simulink model "STM32"  (R2019b)
settings: Solver=FixedStepAuto  StartTime=0.0  StopTime=5  RelTol=1e-3  EnableMultiTasking=on
undefined symbols (not defined in the file): DiscIntNeverNeededParam
libraries: simulink x2, eePwmGenerator x1, pspsim x1
settings Model: SILPILModeSetting=veronly  ExtModeTrigDuration=10  Creator=ahmet  LastModifiedBy=ahmet
settings SolverCC: AlgebraicLoopSolver=LineSearch  PositivePriorityOrder=on  AutoInsertRateTranBlk=on
settings OptimizationCC: EnhancedBackFolding=on  PassReuseOutputArgsAs=Individual arguments  ZeroExternalMemoryAtStartup=off  ZeroInternalMemoryAtStartup=off  MaxStackSize=64  OptimizeBlockOrder=speed  DifferentSizesBufferReuse=on  OptimizationCustomize=off  EfficientTunableParamExpr=on
settings DebuggingCC: AlgebraicLoopMsg=none  ParameterTunabilityLossMsg=error
settings HardwareCC: ProdBitPerPointer=32  ProdBitPerSizeT=32  ProdBitPerPtrDiffT=32  ProdLargestAtomicInteger=Long  ProdLargestAtomicFloat=Double  ProdWordSize=32  ProdHWDeviceType=ARM Compatible->ARM Cortex
settings ModelReferenceCC: ModelReferenceNumInstancesAllowed=Single
settings SFSimCC: MATLABDynamicMemAlloc=off
settings RTWCC: SystemTargetFile=ert.tlc  HardwareBoard=STM32F4-Discovery  TLCOptions="-aInlineSetEventsForThisBaseRateFcn=TLC_FALSE -aSuppressMultiTaskScheduler=TLC_FALSE   -aRateBasedStepFcn=1"  TemplateMakefile=ert_default_tmf  GenerateReport=on  Toolchain=GNU Tools for ARM Embedded Processors  IncludeHyperlinkInReport=on  LaunchReport=on  GenerateTraceInfo=on  GenerateTraceReport=on  GenerateTraceReportSl=on  GenerateTraceReportSf=on  GenerateTraceReportEml=on
settings CodeAppCC: ForceParamTrailComments=on  IgnoreCustomStorageClasses=off  OperatorAnnotations=on  SimulinkDataObjDesc=on  SFDataObjDesc=on  InsertBlockDesc=on
settings ERTTargetCC: CodeReplacementLibrary=ARM Cortex-M (Optimized)  ExtModeStaticAllocSize=2000

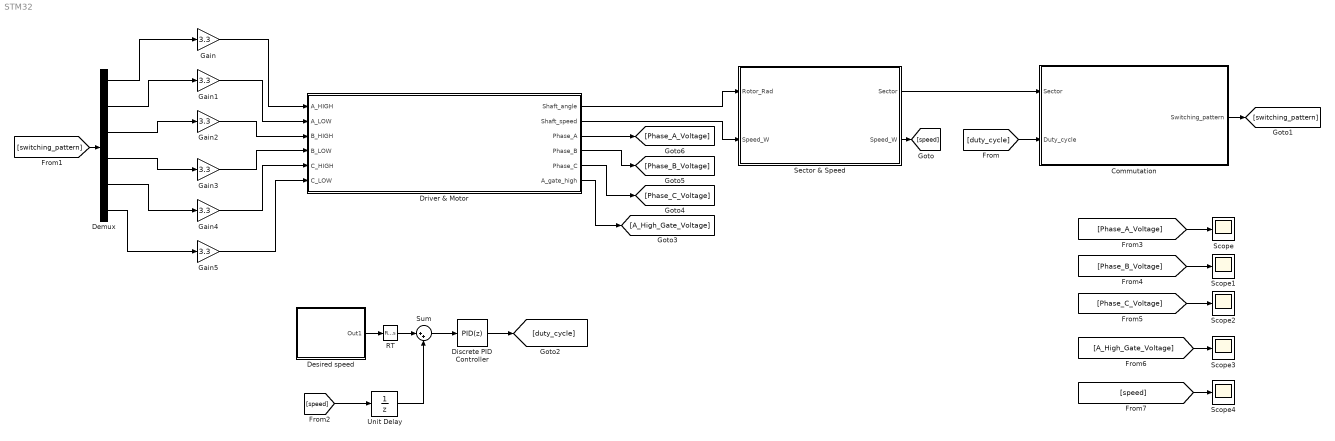
== system STM32 ==
  Commutation : Subsystem
  Demux : Demux  Outputs=6
  "Desired speed " : Subsystem
  Discrete PID Controller : simulink/Continuous/PID Controller  Controller=PID  Form=Parallel  TimeDomain=Discrete-time  SampleTime=10000e-05  IntegratorMethod=Forward Euler  FilterMethod=Forward Euler  ControllerParametersSource=internal  P=0.01  I=0.1  D=0  UseFilter=on  N=100  TunerSelectOption=Transfer Function Based (PID Tuner App)  InitialConditionSource=internal  InitialConditionForIntegrator=0  InitialConditionForFilter=0  DifferentiatorICPrevScaledInput=0  ExternalReset=none  TrackingMode=off  Kt=1  LimitOutput=on  UpperSaturationLimit=1  LowerSaturationLimit=0.5  LinearizeAsGain=off  AntiWindupMode=back-calculation  Kb=1  POutMin=[]  POutMax=[]  IOutMin=[]  IOutMax=[]  DOutMin=[]  DOutMax=[]  NOutMin=[]  NOutMax=[]  SumOutMin=[]  SumOutMax=[]  SaturationOutMin=[]  SaturationOutMax=[]  PParamMin=[]  PParamMax=[]  IParamMin=[]  IParamMax=[]  DParamMin=[]  DParamMax=[]  NParamMin=[]  NParamMax=[]  KbParamMin=[]  KbParamMax=[]  KtParamMin=[]  KtParamMax=[]  KbOutMin=[]  KbOutMax=[]  KtOutMin=[]  KtOutMax=[]  IntegratorOutMin=[]  IntegratorOutMax=[]  FilterOutMin=[]  FilterOutMax=[]  SumI1OutMin=[]  SumI1OutMax=[]  SumI2OutMin=[]  SumI2OutMax=[]  SumI3OutMin=[]  SumI3OutMax=[]  SumI4OutMin=[]  SumI4OutMax=[]  SumDOutMin=[]  SumDOutMax=[]  DifferentiatorOutMin=[]  DifferentiatorOutMax=[]  FilterDiffOutCoefMin=[]  FilterDiffOutCoefMax=[]  ReciprocalOutMin=[]  ReciprocalOutMax=[]  SumDenOutMin=[]  SumDenOutMax=[]  SumNumOutMin=[]  SumNumOutMax=[]  DivideOutMin=[]  DivideOutMax=[]  IntegratorContinuousStateAttributes=''  IntegratorStateMustResolveToSignalObject=off  IntegratorRTWStateStorageClass=Auto  FilterContinuousStateAttributes=''  FilterStateMustResolveToSignalObject=off  FilterRTWStateStorageClass=Auto  ParallelPVariant=InternalParameters  IdealPVariant=Disabled  IVariant=InternalParameters  DVariant=InternalParameters  IntegratorVariant=Discrete  SatVariant=Enabled  AWVariant=BackCalculation  PCopyVariant=Disabled  TRVariant=Disabled  FdbkBlocksVariant=Forward  IdealPFdbkVariant=Disabled  SatFdbkVariant=Disabled  DerivativeFilterVariant=ForwardEulerFilter  NVariant=InternalParameters  NCopyVariant=Disabled  FilterICVariant=InternalICsFilter  IntegratorICVariant=InternalICs  ExternalResetVariant=Disabled  TRSumVariant=Passthrough  SumFdbkVariant=Disabled  SumVariant=Sum_PID
  Driver & Motor : Subsystem
  Gain{,1..5} (6 alike) : Gain  Gain=3.3
  RT : RateTransition  OutPortSampleTime=1e-05
  Scope{,1..4} (5 alike) : Scope
  "Sector & Speed " : Subsystem
  Sum : Sum  Inputs=|++
  Unit Delay : UnitDelay  SampleTime=-1  HasFrameUpgradeWarning=on
  wires:
  Driver & Motor/1(Shaft_angle) -> "Sector & Speed "/1(Rotor_Rad)
  Driver & Motor/2("Shaft_speed ") -> "Sector & Speed "/2("Speed_W ")
  "Sector & Speed "/1("Sector ") -> Commutation/1("Sector ")
  "Sector & Speed "/2(Speed_W) -> [speed]
  [duty_cycle] -> Commutation/2("Duty_cycle ")
  Commutation/1("Switching_pattern ") -> [switching_pattern]
  [switching_pattern] -> Demux/1
  Gain/1 -> Driver & Motor/1("A_HIGH ")
  Gain2/1 -> Driver & Motor/3("B_HIGH ")
  Gain3/1 -> Driver & Motor/4("B_LOW ")
  Gain4/1 -> Driver & Motor/5("C_HIGH ")
  Gain1/1 -> Driver & Motor/2("A_LOW ")
  "Desired speed "/1(Out1) -> RT/1
  Sum/1 -> Discrete PID Controller/1
  Discrete PID Controller/1 -> [duty_cycle]
  Demux/1 -> Gain/1
  Demux/6 -> Gain5/1
  Demux/5 -> Gain4/1
  Demux/4 -> Gain3/1
  Demux/3 -> Gain2/1
  Demux/2 -> Gain1/1
  RT/1 -> Sum/1
  [speed] -> Unit Delay/1
  Unit Delay/1 -> Sum/2
  Gain5/1 -> Driver & Motor/6("C_LOW ")
  Driver & Motor/6("A_gate_high ") -> [A_High_Gate_Voltage]
  Driver & Motor/5(Phase_C) -> [Phase_C_Voltage]
  Driver & Motor/4("Phase_B ") -> [Phase_B_Voltage]
  Driver & Motor/3("Phase_A ") -> [Phase_A_Voltage]
  [Phase_A_Voltage] -> Scope/1
  [Phase_B_Voltage] -> Scope1/1
  [Phase_C_Voltage] -> Scope2/1
  [A_High_Gate_Voltage] -> Scope3/1
  [speed] -> Scope4/1

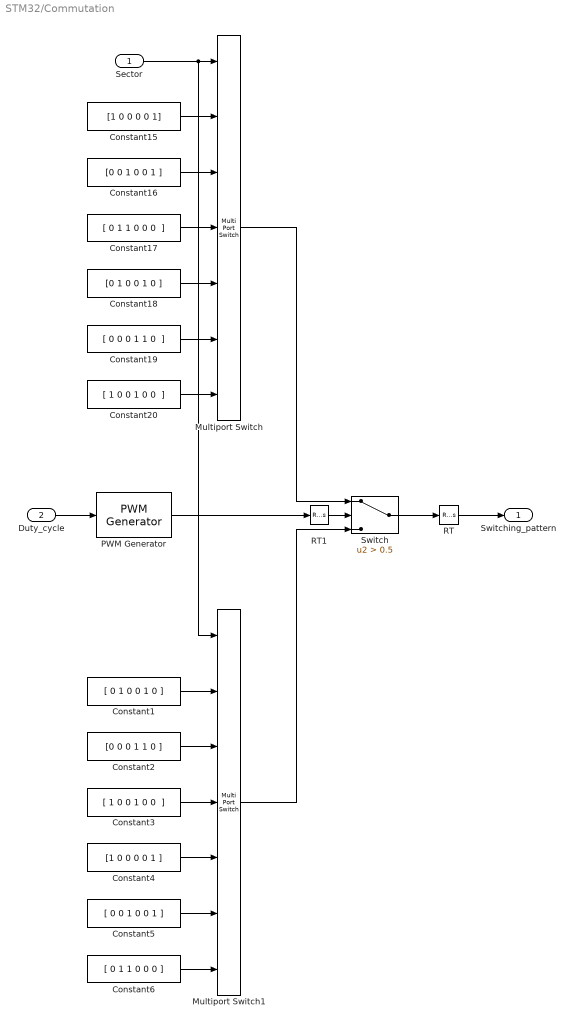
== system STM32/Commutation ==
  "Sector " : Inport
  "Duty_cycle " : Inport  Port=2
  Constant1 : Constant  Value=[ 0 1 0 0 1 0 ]
  Constant15 : Constant  Value=[1 0 0 0 0 1]
  Constant16 : Constant  Value=[0 0 1 0 0 1 ]
  Constant17 : Constant  Value="[ 0 1 1 0 0 0  ]"
  Constant18 : Constant  Value=[0 1 0 0 1 0 ]
  Constant19 : Constant  Value="[ 0 0 0 1 1 0  ]"
  Constant2 : Constant  Value=[0 0 0 1 1 0 ]
  Constant20 : Constant  Value="[ 1 0 0 1 0 0  ]"
  Constant3 : Constant  Value="[ 1 0 0 1 0 0  ]"
  Constant4 : Constant  Value=[1 0 0 0 0 1 ]
  Constant5 : Constant  Value=[ 0 0 1 0 0 1 ]
  Constant6 : Constant  Value=[ 0 1 1 0 0 0 ]
  Multiport Switch : MultiPortSwitch  Inputs=6
  Multiport Switch1 : MultiPortSwitch  Inputs=6
  PWM Generator : eePwmGenerator/PWM Generator  CarrCount=Up  Tper=1000  Ts=10000e-05
      settings: SourceProductName=Simscape Electrical
  RT : RateTransition  Deterministic=off  OutPortSampleTime=5e-05
  RT1 : RateTransition  OutPortSampleTime=2e-05
  Switch : Switch  Criteria=u2 > Threshold  Threshold=0.5
  "Switching_pattern " : Outport
  wires:
  RT/1 -> "Switching_pattern "/1
  Constant19/1 -> Multiport Switch/6
  Constant2/1 -> Multiport Switch1/3
  PWM Generator/1 -> RT1/1
  Constant4/1 -> Multiport Switch1/5
  Constant6/1 -> Multiport Switch1/7
  Constant3/1 -> Multiport Switch1/4
  Multiport Switch1/1 -> Switch/3
  Constant20/1 -> Multiport Switch/7
  Constant5/1 -> Multiport Switch1/6
  Constant1/1 -> Multiport Switch1/2
  "Sector "/1 -> Multiport Switch1/1, Multiport Switch/1
  Constant17/1 -> Multiport Switch/4
  "Duty_cycle "/1 -> PWM Generator/1
  Multiport Switch/1 -> Switch/1
  Constant18/1 -> Multiport Switch/5
  Constant15/1 -> Multiport Switch/2
  Constant16/1 -> Multiport Switch/3
  Switch/1 -> RT/1
  RT1/1 -> Switch/2

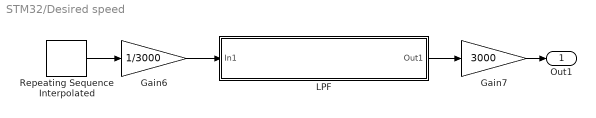
== system STM32/Desired speed  ==
  Gain6 : Gain  Gain=1/3000
  Gain7 : Gain  Gain=3000
  "LPF " : Subsystem
  Repeating Sequence Interpolated : simulink/Sources/Repeating Sequence Interpolated  OutValues=[0 1025/2 1025/2 1025 1025 2050 2050 2050]  TimeValues=[0 10 20 30 40 50 60 70]/2  LookUpMeth=Interpolation-Use End Values  tsamp=10000e-05  OutMin=[]  OutMax=[]  OutDataTypeStr=double  OutputDataTypeScalingMode=double  OutDataType=fixdt(0,8)  OutScaling=2^-10
  Out1 : Outport
  wires:
  Gain6/1 -> "LPF "/1(In1)
  Gain7/1 -> Out1/1
  Repeating Sequence Interpolated/1 -> Gain6/1
  "LPF "/1(Out1) -> Gain7/1

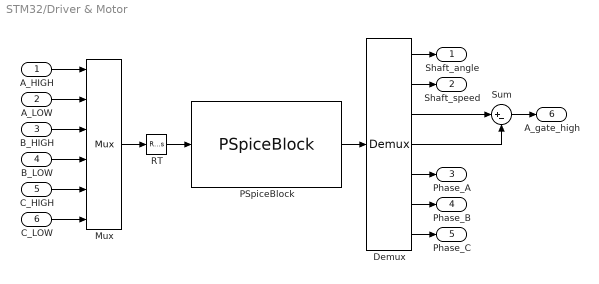
== system STM32/Driver & Motor ==
  "A_HIGH " : Inport
  "A_LOW " : Inport  Port=2
  "B_HIGH " : Inport  Port=3
  "B_LOW " : Inport  Port=4
  "C_HIGH " : Inport  Port=5
  "C_LOW " : Inport  Port=6
  Demux : Demux  Outputs=7
  Mux : Mux  Inputs=6
      settings: DisplayOption=signals
  PSpiceBlock : pspsim/PSpiceBlock  SFunctionModules=''
      settings: SourceProductName=PSpice Block
  RT : RateTransition  OutPortSampleTime=1e-05
  Sum : Sum  Inputs=|+-
  Shaft_angle : Outport
  "Shaft_speed " : Outport  Port=2
  "Phase_A " : Outport  Port=3
  "Phase_B " : Outport  Port=4
  Phase_C : Outport  Port=5
  "A_gate_high " : Outport  Port=6
  wires:
  "B_LOW "/1 -> Mux/4
  "B_HIGH "/1 -> Mux/3
  "C_HIGH "/1 -> Mux/5
  "A_HIGH "/1 -> Mux/1
  "A_LOW "/1 -> Mux/2
  "C_LOW "/1 -> Mux/6
  Mux/1 -> RT/1
  PSpiceBlock/1 -> Demux/1
  Demux/1 -> Shaft_angle/1
  Demux/2 -> "Shaft_speed "/1
  RT/1 -> PSpiceBlock/1
  Demux/7 -> Phase_C/1
  Demux/6 -> "Phase_B "/1
  Demux/5 -> "Phase_A "/1
  Demux/4 -> Sum/2
  Demux/3 -> Sum/1
  Sum/1 -> "A_gate_high "/1

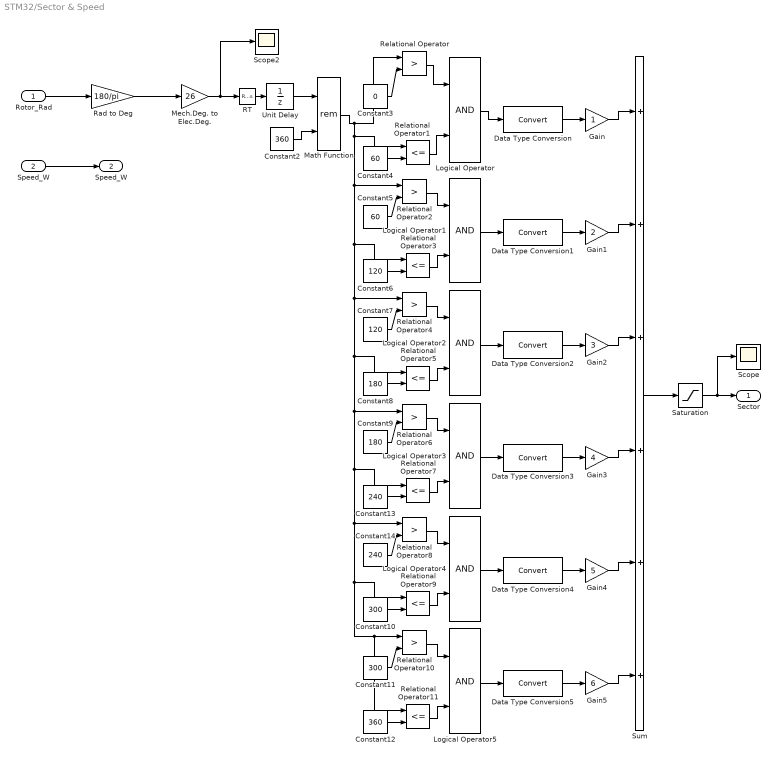
== system STM32/Sector & Speed  ==
  Rotor_Rad : Inport
  "Speed_W " : Inport  Port=2
  Constant10 : Constant  Value=300
  Constant11 : Constant  Value=300
  Constant12 : Constant  Value=360
  Constant13 : Constant  Value=240
  Constant14 : Constant  Value=240
  Constant2 : Constant  Value=360
  Constant3 : Constant  Value=0
  Constant4 : Constant  Value=60
  Constant5 : Constant  Value=60
  Constant6 : Constant  Value=120
  Constant7 : Constant  Value=120
  Constant8 : Constant  Value=180
  Constant9 : Constant  Value=180
  Data Type Conversion{,1..5} (6 alike) : DataTypeConversion
  Gain : Gain
  Gain1 : Gain  Gain=2
  Gain2 : Gain  Gain=3
  Gain3 : Gain  Gain=4
  Gain4 : Gain  Gain=5
  Gain5 : Gain  Gain=6
  Logical Operator{,1..5} (6 alike) : Logic  AllPortsSameDT=off  OutDataTypeStr=boolean
  Math Function : Math  Operator=rem  SignedPower=off  SaturateOnIntegerOverflow=on
  Mech.Deg. to Elec.Deg. : Gain  Gain=26
  RT : RateTransition  OutPortSampleTime=2e-05
  "Rad to Deg " : Gain  Gain=180/pi
  Relational Operator{,2,4,6,8,10} (6 alike) : RelationalOperator  Operator=>  OutDataTypeStr=boolean  RndMeth=Simplest
  Relational Operator{1,3,5,7,9,11} (6 alike) : RelationalOperator  Operator=<=  OutDataTypeStr=boolean  RndMeth=Simplest
  Saturation : Saturate  UpperLimit=6  LowerLimit=1
  Scope : Scope
  Scope2 : Scope
  Sum : Sum  Inputs=++++++
  Unit Delay : UnitDelay  SampleTime=2e-5  HasFrameUpgradeWarning=on
  "Sector " : Outport
  Speed_W : Outport  Port=2
  wires:
  Data Type Conversion3/1 -> Gain3/1
  Relational Operator7/1 -> Logical Operator3/2
  Logical Operator4/1 -> Data Type Conversion4/1
  Constant6/1 -> Relational Operator3/2
  Relational Operator/1 -> Logical Operator/1
  Data Type Conversion5/1 -> Gain5/1
  "Rad to Deg "/1 -> Mech.Deg. to Elec.Deg./1
  Constant5/1 -> Relational Operator2/2
  Math Function/1 -> Relational Operator/1, Relational Operator6/1, Relational Operator11/1, Relational Operator10/1, Relational Operator9/1, Relational Operator8/1, Relational Operator7/1, Relational Operator5/1, Relational Operator4/1, Relational Operator3/1, Relational Operator2/1, Relational Operator1/1
  Relational Operator11/1 -> Logical Operator5/2
  Relational Operator10/1 -> Logical Operator5/1
  Gain4/1 -> Sum/5
  Constant14/1 -> Relational Operator8/2
  Mech.Deg. to Elec.Deg./1 -> RT/1, Scope2/1
  Gain3/1 -> Sum/4
  Data Type Conversion2/1 -> Gain2/1
  Saturation/1 -> "Sector "/1, Scope/1
  Relational Operator8/1 -> Logical Operator4/1
  Constant3/1 -> Relational Operator/2
  Constant2/1 -> Math Function/2
  Unit Delay/1 -> Math Function/1
  Constant10/1 -> Relational Operator9/2
  Relational Operator3/1 -> Logical Operator1/2
  Logical Operator1/1 -> Data Type Conversion1/1
  Relational Operator5/1 -> Logical Operator2/2
  Relational Operator2/1 -> Logical Operator1/1
  Data Type Conversion4/1 -> Gain4/1
  Rotor_Rad/1 -> "Rad to Deg "/1
  Constant12/1 -> Relational Operator11/2
  Gain2/1 -> Sum/3
  Logical Operator3/1 -> Data Type Conversion3/1
  Logical Operator/1 -> Data Type Conversion/1
  Data Type Conversion1/1 -> Gain1/1
  Sum/1 -> Saturation/1
  Constant7/1 -> Relational Operator4/2
  Logical Operator2/1 -> Data Type Conversion2/1
  Relational Operator9/1 -> Logical Operator4/2
  Relational Operator4/1 -> Logical Operator2/1
  Logical Operator5/1 -> Data Type Conversion5/1
  Constant4/1 -> Relational Operator1/2
  Gain5/1 -> Sum/6
  Constant8/1 -> Relational Operator5/2
  Constant13/1 -> Relational Operator7/2
  Relational Operator1/1 -> Logical Operator/2
  Constant11/1 -> Relational Operator10/2
  Gain/1 -> Sum/1
  Gain1/1 -> Sum/2
  Constant9/1 -> Relational Operator6/2
  Data Type Conversion/1 -> Gain/1
  Relational Operator6/1 -> Logical Operator3/1
  "Speed_W "/1 -> Speed_W/1
  RT/1 -> Unit Delay/1

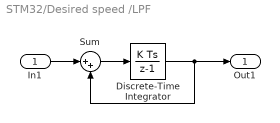
== system STM32/Desired speed /LPF  ==
  In1 : Inport
  Discrete-Time Integrator : DiscreteIntegrator  gainval=20  SampleTime=10000e-05  ICPrevOutput=DiscIntNeverNeededParam  ICPrevScaledInput=DiscIntNeverNeededParam
  Sum : Sum  Inputs=|++
  Out1 : Outport
  wires:
  In1/1 -> Sum/1
  Sum/1 -> Discrete-Time Integrator/1
  Discrete-Time Integrator/1 -> Out1/1, Sum/2
